simulink model "model_linearization"  (R2015b)
settings: Solver=ode3  StartTime=0.0  StopTime=inf  FixedStep=0.01  RelTol=1e-3
libraries: aerolib6dof2 x1
settings Model: Creator=rcasado  LastModifiedBy=rcasado
settings DataIOCC: SaveFormat=Array
settings DebuggingCC: MultiTaskRateTransMsg=warning
settings HardwareCC: ProdBitPerPointer=32  ProdLargestAtomicFloat=None  ProdIntDivRoundTo=Undefined  ProdEndianess=Unspecified  ProdWordSize=32  ProdHWDeviceType=32-bit Generic
settings GRTTargetCC: GeneratePreprocessorConditionals=Disable all
settings ConfigComp: CovModelRefEnable=Off

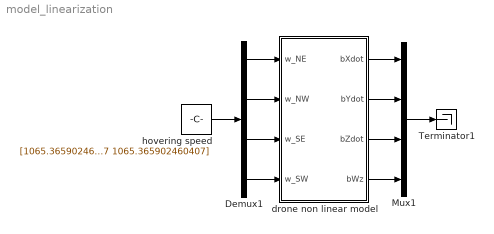
== system model_linearization ==
  Demux1 : Demux
  Mux1 : Mux
  Terminator1 : Terminator
  drone non linear model : Subsystem
  hovering speed : Constant  Value=[1065.365902460407 1065.365902460407 1065.365902460407 1065.365902460407]
  wires:
  Demux1/3 -> drone non linear model/3(w_SE)
  Demux1/2 -> drone non linear model/2(w_NW)
  Mux1/1 -> Terminator1/1
  hovering speed/1 -> Demux1/1
  drone non linear model/1(bXdot) -> Mux1/1
  drone non linear model/3(bZdot) -> Mux1/3
  drone non linear model/2(bYdot) -> Mux1/2
  Demux1/4 -> drone non linear model/4(w_SW)
  Demux1/1 -> drone non linear model/1(w_NE)
  drone non linear model/4(bWz) -> Mux1/4

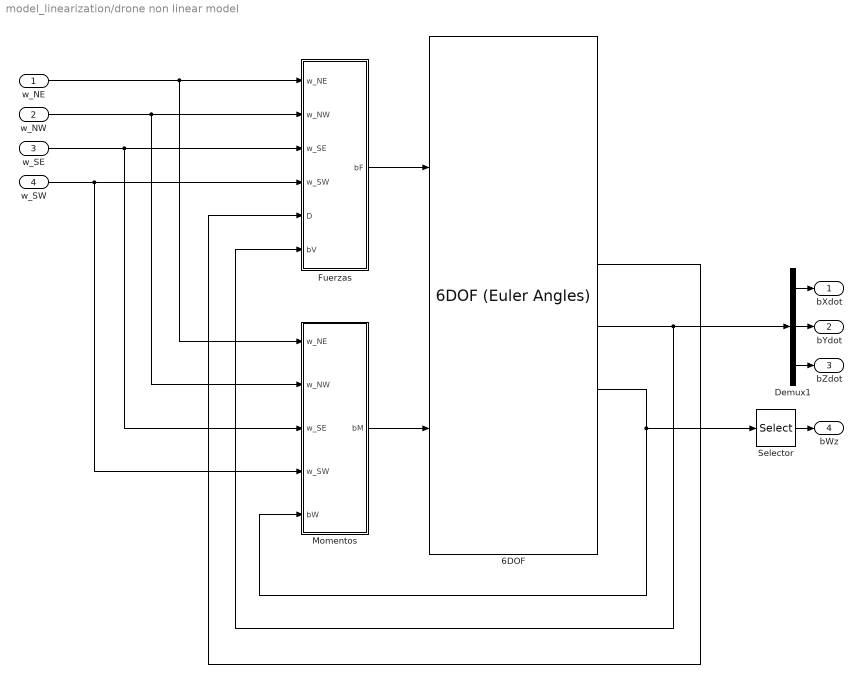
== system model_linearization/drone non linear model ==
  w_NE : Inport
  w_NW : Inport  Port=2
  w_SE : Inport  Port=3
  w_SW : Inport  Port=4
  6DOF : aerolib6dof2/6DOF (Euler Angles)  units=Metric (MKS)  mtype=Fixed  rep=Euler Angles  xme_0=[0 0 0]  Vm_0=[0 0 0]  eul_0=[0 0 0]  pm_0=[0 0 0]  mass_0=1.840  mass_e=0.5  mass_f=2.0  inertia="[0.024916667  0  0 ; 0 0.024916667 0 ; 0 0 0.049066667]"  inertia_e=eye(3)  inertia_f=2*eye(3)  k_quat=1.0  vre_flag=on
  Demux1 : Demux  Outputs=3
  Fuerzas : Subsystem
  Momentos : Subsystem
  Selector : Selector  InputPortWidth=3  IndexOptions=Index vector (dialog)  Indices=[3]  OutputSizes=1
  bXdot : Outport
  bYdot : Outport  Port=2
  bZdot : Outport  Port=3
  bWz : Outport  Port=4
  wires:
  Momentos/1(bM) -> 6DOF/2
  w_NE/1 -> Momentos/1(w_NE), Fuerzas/1(w_NE)
  w_NW/1 -> Momentos/2(w_NW), Fuerzas/2(w_NW)
  w_SE/1 -> Momentos/3(w_SE), Fuerzas/3(w_SE)
  w_SW/1 -> Momentos/4(w_SW), Fuerzas/4(w_SW)
  6DOF/4 -> Fuerzas/5(D)
  Fuerzas/1(bF) -> 6DOF/1
  6DOF/6 -> Momentos/5(bW), Selector/1
  6DOF/5 -> Fuerzas/6(bV), Demux1/1
  Demux1/1 -> bXdot/1
  Demux1/2 -> bYdot/1
  Demux1/3 -> bZdot/1
  Selector/1 -> bWz/1

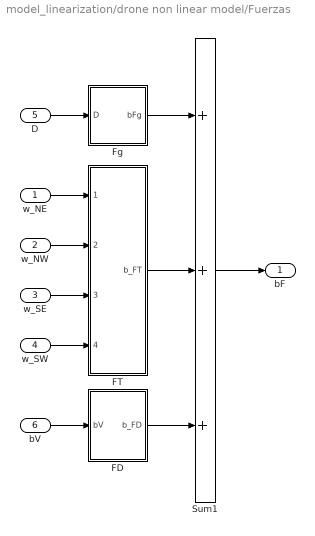
== system model_linearization/drone non linear model/Fuerzas ==
  w_NE : Inport
  w_NW : Inport  Port=2
  w_SE : Inport  Port=3
  w_SW : Inport  Port=4
  D : Inport  Port=5
  bV : Inport  Port=6
  FD : Subsystem
  FT : Subsystem
  Fg : Subsystem
  Sum1 : Sum  Inputs=+++
  bF : Outport
  wires:
  D/1 -> Fg/1(D)
  Fg/1(bFg) -> Sum1/1
  FT/1(b_FT) -> Sum1/2
  w_SW/1 -> FT/4(w_SW)
  w_NE/1 -> FT/1(w_NE)
  w_SE/1 -> FT/3(w_SE)
  w_NW/1 -> FT/2(w_NW)
  Sum1/1 -> bF/1
  bV/1 -> FD/1(bV)
  FD/1(b_FD) -> Sum1/3

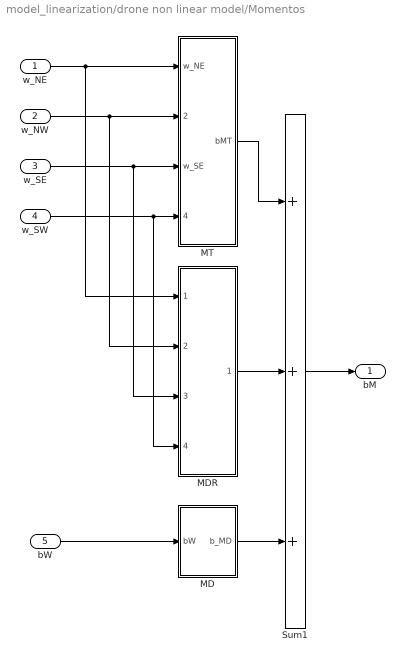
== system model_linearization/drone non linear model/Momentos ==
  w_NE : Inport
  w_NW : Inport  Port=2
  w_SE : Inport  Port=3
  w_SW : Inport  Port=4
  bW : Inport  Port=5
  MD : Subsystem
  MDR : Subsystem
  MT : Subsystem
  Sum1 : Sum  Inputs=+++
  bM : Outport
  wires:
  bW/1 -> MD/1(bW)
  MT/1(bMT) -> Sum1/1
  w_SW/1 -> MT/4(w_SW), MDR/4(w_SW)
  w_NE/1 -> MT/1(w_NE), MDR/1(w_NE)
  w_SE/1 -> MT/3(w_SE), MDR/3(w_SE)
  w_NW/1 -> MT/2(w_NW), MDR/2(w_NW)
  Sum1/1 -> bM/1
  MD/1(b_MD) -> Sum1/3
  MDR/1(b_MDR) -> Sum1/2

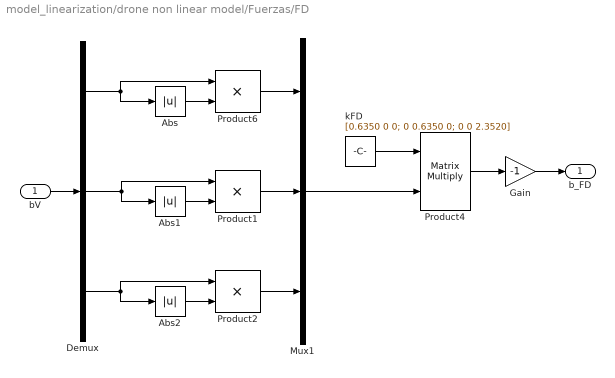
== system model_linearization/drone non linear model/Fuerzas/FD ==
  bV : Inport
  Abs : Abs
  Abs1 : Abs
  Abs2 : Abs
  Demux : Demux  Outputs=3
  Gain : Gain  Gain=-1
  Mux1 : Mux  Inputs=3
  Product1 : Product
  Product2 : Product
  Product4 : Product  Multiplication=Matrix(*)
  Product6 : Product
  kFD : Constant  Value=[0.6350 0 0; 0 0.6350 0; 0 0 2.3520]
  b_FD : Outport
  wires:
  kFD/1 -> Product4/1
  Product4/1 -> Gain/1
  Mux1/1 -> Product4/2
  Product1/1 -> Mux1/2
  bV/1 -> Demux/1
  Abs/1 -> Product6/2
  Abs1/1 -> Product1/2
  Abs2/1 -> Product2/2
  Demux/1 -> Product6/1, Abs/1
  Demux/2 -> Product1/1, Abs1/1
  Demux/3 -> Product2/1, Abs2/1
  Product6/1 -> Mux1/1
  Product2/1 -> Mux1/3
  Gain/1 -> b_FD/1

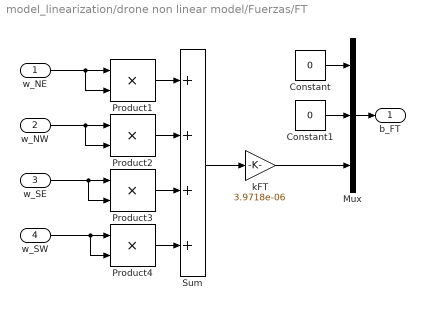
== system model_linearization/drone non linear model/Fuerzas/FT ==
  w_NE : Inport
  w_NW : Inport  Port=2
  w_SE : Inport  Port=3
  w_SW : Inport  Port=4
  Constant : Constant  Value=0
  Constant1 : Constant  Value=0
  Mux : Mux  Inputs=3
  Product{1..4} (4 alike) : Product
  Sum : Sum  Inputs=++++
  kFT : Gain  Gain=3.9718e-06
  b_FT : Outport
  wires:
  Product4/1 -> Sum/4
  Product3/1 -> Sum/3
  Product2/1 -> Sum/2
  w_NW/1 -> Product2/2, Product2/1
  w_NE/1 -> Product1/2, Product1/1
  Product1/1 -> Sum/1
  Mux/1 -> b_FT/1
  w_SE/1 -> Product3/2, Product3/1
  w_SW/1 -> Product4/2, Product4/1
  Sum/1 -> kFT/1
  Constant/1 -> Mux/1
  Constant1/1 -> Mux/2
  kFT/1 -> Mux/3

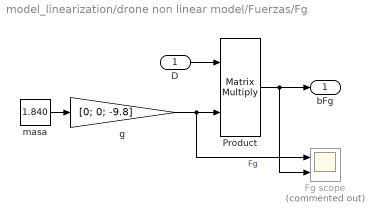
== system model_linearization/drone non linear model/Fuerzas/Fg ==
  D : Inport
  Fg scope : Scope  Commented=on  NumInputPorts=2
  Product : Product  Multiplication=Matrix(*)
  g : Gain  Gain=[0; 0; -9.8]
  masa : Constant  Value=1.840
  bFg : Outport
  wires:
  Product/1 -> Fg scope/2, bFg/1
  D/1 -> Product/1
  masa/1 -> g/1
  g/1 -> Fg scope/1, Product/2  "Fg"

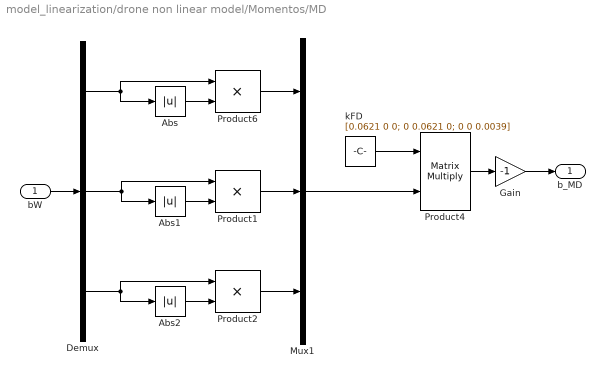
== system model_linearization/drone non linear model/Momentos/MD ==
  bW : Inport
  Abs : Abs
  Abs1 : Abs
  Abs2 : Abs
  Demux : Demux  Outputs=3
  Gain : Gain  Gain=-1
  Mux1 : Mux  Inputs=3
  Product1 : Product
  Product2 : Product
  Product4 : Product  Multiplication=Matrix(*)
  Product6 : Product
  kFD : Constant  Value=[0.0621 0 0; 0 0.0621 0; 0 0 0.0039]
  b_MD : Outport
  wires:
  kFD/1 -> Product4/1
  Product4/1 -> Gain/1
  Mux1/1 -> Product4/2
  Product1/1 -> Mux1/2
  bW/1 -> Demux/1
  Abs/1 -> Product6/2
  Abs1/1 -> Product1/2
  Abs2/1 -> Product2/2
  Demux/1 -> Product6/1, Abs/1
  Demux/2 -> Product1/1, Abs1/1
  Demux/3 -> Product2/1, Abs2/1
  Product6/1 -> Mux1/1
  Product2/1 -> Mux1/3
  Gain/1 -> b_MD/1

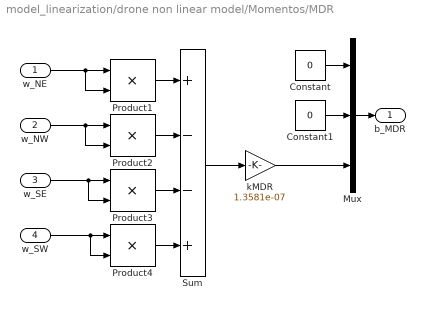
== system model_linearization/drone non linear model/Momentos/MDR ==
  w_NE : Inport
  w_NW : Inport  Port=2
  w_SE : Inport  Port=3
  w_SW : Inport  Port=4
  Constant : Constant  Value=0
  Constant1 : Constant  Value=0
  Mux : Mux  Inputs=3
  Product{1..4} (4 alike) : Product
  Sum : Sum  Inputs=+--+
  kMDR : Gain  Gain=1.3581e-07
  b_MDR : Outport
  wires:
  Product4/1 -> Sum/4
  Product3/1 -> Sum/3
  Product2/1 -> Sum/2
  w_NW/1 -> Product2/2, Product2/1
  w_NE/1 -> Product1/2, Product1/1
  Product1/1 -> Sum/1
  Mux/1 -> b_MDR/1
  w_SE/1 -> Product3/2, Product3/1
  w_SW/1 -> Product4/2, Product4/1
  Sum/1 -> kMDR/1
  Constant/1 -> Mux/1
  Constant1/1 -> Mux/2
  kMDR/1 -> Mux/3

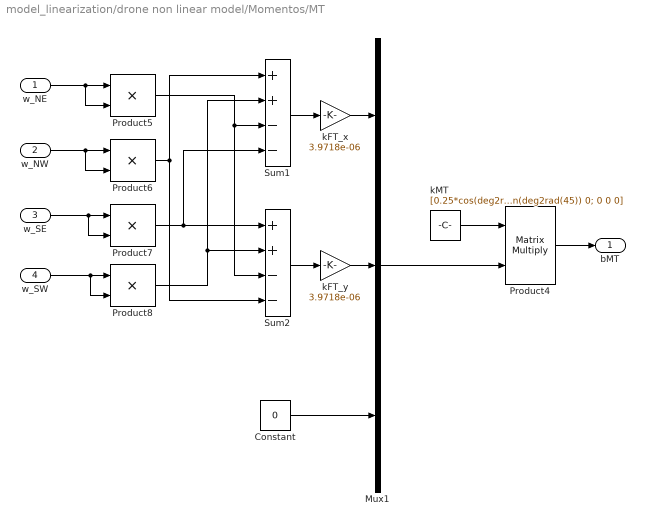
== system model_linearization/drone non linear model/Momentos/MT ==
  w_NE : Inport
  w_NW : Inport  Port=2
  w_SE : Inport  Port=3
  w_SW : Inport  Port=4
  Constant : Constant  Value=0
  Mux1 : Mux  Inputs=3
  Product4 : Product  Multiplication=Matrix(*)
  Product{5..8} (4 alike) : Product
  Sum1 : Sum  Inputs=++--
  Sum2 : Sum  Inputs=++--
  kFT_x : Gain  Gain=3.9718e-06
  kFT_y : Gain  Gain=3.9718e-06
  kMT : Constant  Value=[0.25*cos(deg2rad(45)) 0 0; 0 0.25*sin(deg2rad(45)) 0; 0 0 0]
  bMT : Outport
  wires:
  kMT/1 -> Product4/1
  Product4/1 -> bMT/1
  Product8/1 -> Sum1/2, Sum2/2
  Product7/1 -> Sum2/1, Sum1/4
  w_NW/1 -> Product6/2, Product6/1
  w_NE/1 -> Product5/2, Product5/1
  Product6/1 -> Sum2/4, Sum1/1
  Mux1/1 -> Product4/2
  w_SE/1 -> Product7/2, Product7/1
  w_SW/1 -> Product8/2, Product8/1
  kFT_y/1 -> Mux1/2
  Sum1/1 -> kFT_x/1
  Sum2/1 -> kFT_y/1
  Product5/1 -> Sum2/3, Sum1/3
  kFT_x/1 -> Mux1/1
  Constant/1 -> Mux1/3
